simulink model "hdl_block"  (R2022b)
settings: Solver=FixedStepDiscrete  StartTime=0.0  StopTime=10.0  RelTol=1e-3
settings Model: DataTypeOverride=Off  Creator=cotti  LastModifiedBy=cotti
settings SolverCC: AlgebraicLoopSolver=TrustRegion
settings DataIOCC: LimitDataPoints=on  SaveOutput=off  SaveTime=off
settings OptimizationCC: BlockReduction=off  ConditionallyExecuteInputs=off  DefaultParameterBehavior=Inlined  LifeSpan=inf
settings DebuggingCC: AlgebraicLoopMsg=error  SingleTaskRateTransMsg=error  UnconnectedInputMsg=warning  UnconnectedOutputMsg=warning  UnconnectedLineMsg=warning  AllowSymbolicDim=off  StrictBusMsg=ErrorOnBusTreatedAsVector  SFUnexpectedBacktrackingDiag=warning  SFNoUnconditionalDefaultTransitionDiag=warning  SFExecutionAtInitializationDiag=none  SFMachineParentedDataDiag=warning  ArithmeticOperatorsInVariantConditions=warning
settings HardwareCC: ProdBitPerPointer=32  ProdBitPerSizeT=32  ProdBitPerPtrDiffT=32  ProdLargestAtomicFloat=None  ProdIntDivRoundTo=Undefined  ProdEndianess=Unspecified  ProdWordSize=32  ProdHWDeviceType=ASIC/FPGA->ASIC/FPGA  ProdEqTarget=off
settings ModelReferenceCC: EnableRefExpFcnMdlSchedulingChecks=on
settings SFSimCC: SimUseLocalCustomCode=off  CustomCodeUndefinedFunction=UseInterfaceOnly
settings RTWCC: RTWUseLocalCustomCode=off
settings CodeAppCC: StateflowObjectComments=on
settings GRTTargetCC: TargetLangStandard=C89/C90 (ANSI)
settings ConfigComp: CovScope=ReferencedModels  CovMetricSettings=dw  CovSaveCumulativeToWorkspaceVar=on  CovSaveSingleToWorkspaceVar=on  CovExternalEMLEnable=off  CovSFcnEnable=off

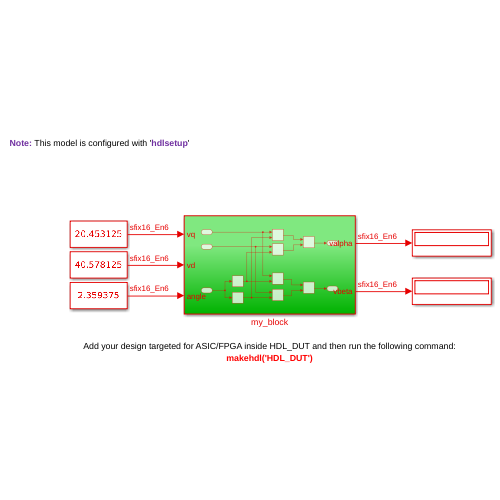
[thumbnail: Simulink's stored preview of the top-level diagram]
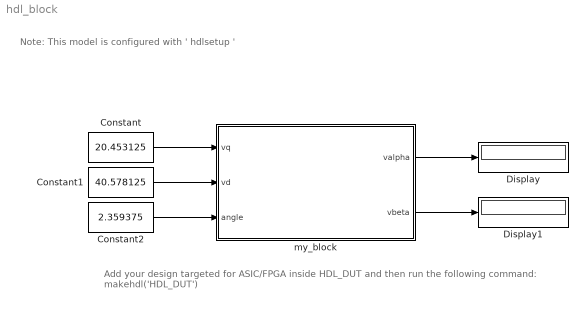
== system hdl_block ==
  note: Note: This model is configured with ' hdlsetup '
  note: Add your design targeted for ASIC/FPGA inside HDL_DUT and then run the following command:
      | makehdl('HDL_DUT')
  Constant : Constant  Value=20.453125  OutDataTypeStr=fixdt(1,16,6)  SampleTime=-1
  Constant1 : Constant  Value=40.578125  OutDataTypeStr=fixdt(1,16,6)  SampleTime=-1
  Constant2 : Constant  Value=2.359375  OutDataTypeStr=fixdt(1,16,6)  SampleTime=-1
  Display : Display
  Display1 : Display
  my_block : Subsystem
  wires:
  Constant/1 -> my_block/1(vq)
  Constant1/1 -> my_block/2(vd)
  Constant2/1 -> my_block/3(angle)
  my_block/1(valpha) -> Display/1
  my_block/2(vbeta) -> Display1/1

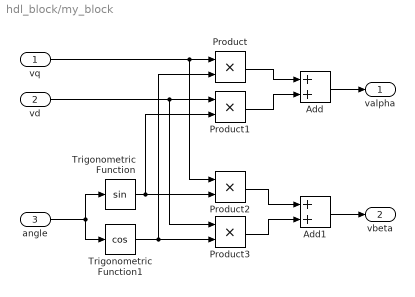
== system hdl_block/my_block ==
  vq : Inport
  vd : Inport  Port=2
  angle : Inport  Port=3
  Add : Sum  OutDataTypeStr=fixdt(1,16,6)
  Add1 : Sum  OutDataTypeStr=fixdt(1,16,6)
  Product{,1..3} (4 alike) : Product
  Trigonometric Function : Trigonometry  ApproximationMethod=CORDIC  NumberOfIterations=1  InterpMethod=Flat
  Trigonometric Function1 : Trigonometry  Operator=cos  ApproximationMethod=CORDIC  NumberOfIterations=1  InterpMethod=Flat
  valpha : Outport  VectorParamsAs1DForOutWhenUnconnected=off
  vbeta : Outport  Port=2  VectorParamsAs1DForOutWhenUnconnected=off
  wires:
  vq/1 -> Product2/1, Product/1
  vd/1 -> Product3/1, Product1/1
  Product1/1 -> Add/2
  Product/1 -> Add/1
  Add/1 -> valpha/1
  Product2/1 -> Add1/1
  Product3/1 -> Add1/2
  Add1/1 -> vbeta/1
  angle/1 -> Trigonometric Function1/1, Trigonometric Function/1
  Trigonometric Function/1 -> Product2/2, Product1/2
  Trigonometric Function1/1 -> Product3/2, Product/2
